simulink model "New_Control_Law"  (R2014a)
settings: configuration reference "AR_Drone_ConfigSet" (kept outside this file)
undefined symbols (not defined in the file or in its folder): Drone_StateModeType, sigbuilder_block
libraries: simulink x8, AR_Drone_2_Library x4
settings Model: SimulationMode=external  ExtModeTrigDuration=48000  Creator=nraman  LastModifiedBy=darenlee

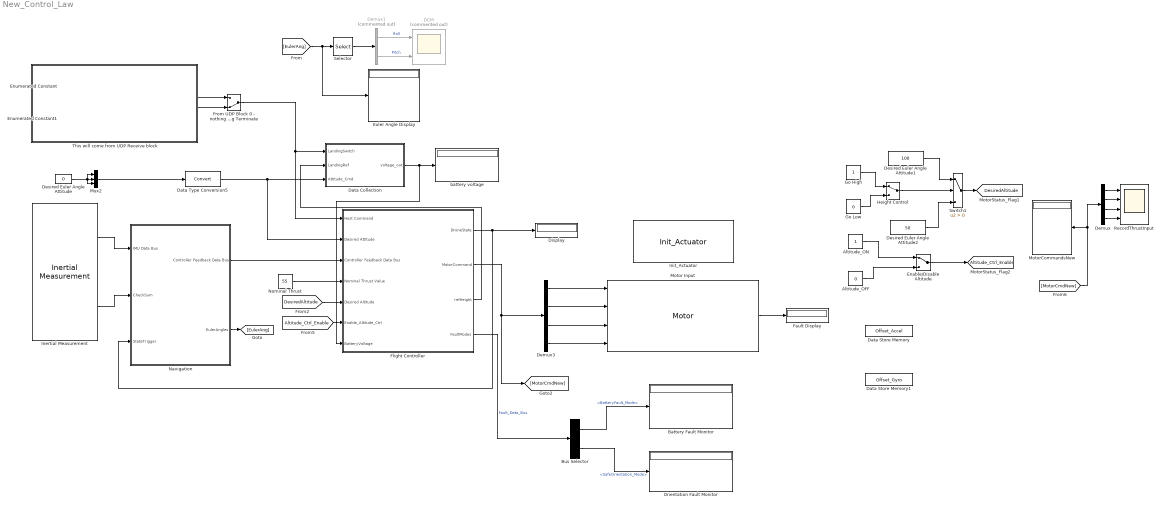
== system New_Control_Law ==
  Altitude_OFF : Constant  Value=0
  Altitude_ON : Constant
  Battery Fault Monitor : Display
  Bus Selector : BusSelector  OutputSignals=BatteryFault_Mode,SafeOrientation_Mode
  DCM : Scope  Commented=on  NumInputPorts=2
      settings: TimeRange=18.24617860016089  YMin=-20~-0.6  YMax=30~0.1  SaveName=EulerAngles
  Data Collection : Subsystem
  Data Store Memory : DataStoreMemory  DataStoreName=Offset_Accel  ReadBeforeWriteMsg=warning  WriteAfterWriteMsg=warning  WriteAfterReadMsg=warning  InitialValue=[0 0]  OutDataTypeStr=double
  Data Store Memory1 : DataStoreMemory  DataStoreName=Offset_Gyro  ReadBeforeWriteMsg=warning  WriteAfterWriteMsg=warning  WriteAfterReadMsg=warning  InitialValue=[0 0 0]  OutDataTypeStr=double
  Data Type Conversion5 : DataTypeConversion
  Demux : Demux
  Demux1 : Demux  Commented=on  Outputs=2
  Demux3 : Demux
  Desired Euler Angle Attitude : Constant  Value=0
  Desired Euler Angle Attitude1 : Constant  Value=100
  Desired Euler Angle Attitude2 : Constant  Value=50
  Display : Display
  Enable/Disable Altitude : ManualSwitch
  Enumerated Constant : simulink/Sources/Enumerated Constant  OutDataTypeStr=Enum: Drone_StateModeType  Value=Drone_StateModeType.Controlled_Flight  SampleTime=inf
  Enumerated Constant1 : simulink/Sources/Enumerated Constant  OutDataTypeStr=Enum: Drone_StateModeType  Value=Drone_StateModeType.Landing_Sequence  SampleTime=inf
  Euler Angle Display : Display
  Fault Display : Display
  Flight Controller : Subsystem
  "From UDP Block 0 - nothing 1 - Initialize 2 - take-off 3 - Land 4 - Landing Terminate " : ManualSwitch  CurrentSetting=0
  Go High : Constant
  Go Low : Constant  Value=0
  Height Control : ManualSwitch
  Inertial Measurement : AR_Drone_2_Library/Inertial Measurement  Ts=1/400
  Init_Actuator : AR_Drone_2_Library/Init_Actuator  ShowSpec=on
  Motor Input : AR_Drone_2_Library/Motor
  MotorCommandsNew : Display
  Mux2 : Mux  Inputs=3
  Navigation : Subsystem
  Nominal Thrust : Constant  Value=55
  Orientation Fault Monitor : Display
  RecordThrustInput : Scope  NumInputPorts=4
      settings: TimeRange=44.32823813354787  YMin=20~20~-5~-5  YMax=85~90~5~5  SaveName=Control_Input
  Selector : Selector  InputPortWidth=3  Indices=[1 2]
  Switch1 : Switch  Criteria=u2 > Threshold
  This will come from UDP Receive block : Subsystem
  battery voltage : Display
  tag scope: Altitude_Ctrl_Enable=global, DesiredAltitude=global
  wires:
  Motor Input/1 -> Fault Display/1
  Data Collection/1(voltage_out) -> Flight Controller/7(BatteryVoltage), battery voltage/1
  Mux2/1 -> Data Type Conversion5/1
  Demux3/1 -> Motor Input/1
  Demux3/2 -> Motor Input/2
  Demux3/3 -> Motor Input/3
  Demux3/4 -> Motor Input/4
  Inertial Measurement/1 -> Navigation/1(IMU Data Bus)
  Inertial Measurement/2 -> Navigation/2(CheckSum)
  Data Type Conversion5/1 -> Flight Controller/2(Desired Attitude), Data Collection/3(Attitude_Cmd)
  Nominal Thrust/1 -> Flight Controller/4(Nominal Thrust Value)
  Navigation/1(Controller Feedback Data Bus) -> Flight Controller/3(Controller Feedback Data Bus)
  Navigation/2(EulerAngles) -> [EulerAng]
  Go High/1 -> Height Control/1
  Go Low/1 -> Height Control/2
  Height Control/1 -> Switch1/2
  Desired Euler Angle Attitude1/1 -> Switch1/1
  Desired Euler Angle Attitude2/1 -> Switch1/3
  Switch1/1 -> [DesiredAltitude]
  [DesiredAltitude] -> Flight Controller/5(Desired Altitude)
  [Altitude_Ctrl_Enable] -> Flight Controller/6(Enable_Altitude_Ctrl)
  Altitude_ON/1 -> Enable/Disable Altitude/1
  Altitude_OFF/1 -> Enable/Disable Altitude/2
  Enable/Disable Altitude/1 -> [Altitude_Ctrl_Enable]
  Enumerated Constant1/1 -> "From UDP Block 0 - nothing 1 - Initialize 2 - take-off 3 - Land 4 - Landing Terminate "/2
  "From UDP Block 0 - nothing 1 - Initialize 2 - take-off 3 - Land 4 - Landing Terminate "/1 -> Flight Controller/1(Host Command), Data Collection/1(LandingSwitch)
  Flight Controller/1(DroneState) -> Navigation/3(StateTrigger), Display/1
  Demux1/1 -> DCM/1  "Roll"
  Demux1/2 -> DCM/2  "Pitch"
  [EulerAng] -> Selector/1, Euler Angle Display/1
  Selector/1 -> Demux1/1
  Enumerated Constant/1 -> "From UDP Block 0 - nothing 1 - Initialize 2 - take-off 3 - Land 4 - Landing Terminate "/1
  Flight Controller/3(refHeight) -> Data Collection/2(LandingRef)
  [MotorCmdNew] -> MotorCommandsNew/1, Demux/1
  Demux/1 -> RecordThrustInput/1
  Demux/2 -> RecordThrustInput/2
  Demux/3 -> RecordThrustInput/3
  Demux/4 -> RecordThrustInput/4
  Flight Controller/2(MotorCommand) -> Demux3/1, [MotorCmdNew]
  Desired Euler Angle Attitude/1 -> Mux2/3, Mux2/2, Mux2/1
  Flight Controller/4(FaultModes) -> Bus Selector/1  "Fault_Data_Bus"
  Bus Selector/1 -> Battery Fault Monitor/1  "<BatteryFault_Mode>"
  Bus Selector/2 -> Orientation Fault Monitor/1  "<SafeOrientation_Mode>"

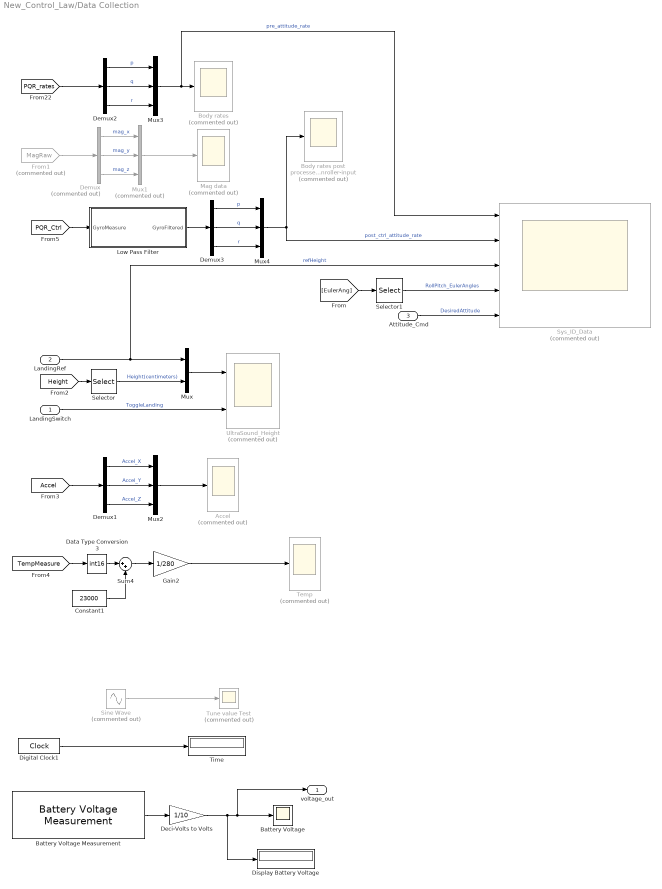
== system New_Control_Law/Data Collection ==
  LandingSwitch : Inport
  LandingRef : Inport  Port=2
  Attitude_Cmd : Inport  Port=3
  Accel : Scope  Commented=on
      settings: ShowLegends=on  TimeRange=100  YMin=1850  YMax=2750  SaveName=Accel
  Battery Voltage : Scope
      settings: YMin=11.935  YMax=12.005  SaveName=RecordedBattery
  Battery Voltage Measurement : AR_Drone_2_Library/Battery Voltage Measurement  SFunctionSpec=void BatteryMeasure_step(single y1[1])  SampleTime=1/400
  Body rates : Scope  Commented=on
      settings: ShowLegends=on  TimeRange=90  YMin=-1000  YMax=1200  SaveName=Gyro
  Body rates post processed - pre-conroller-input : Scope  Commented=on
      settings: ShowLegends=on  TimeRange=90  YMin=-1000  YMax=1200  SaveName=Gyro_PostProcessed
  Constant1 : Constant  Value=23000  OutDataTypeStr=int16
  Data Type Conversion3 : DataTypeConversion  OutDataTypeStr=int16
  Deci-Volts to Volts : Gain  Gain=1/10
  Demux : Demux  Commented=on  Outputs=3
  Demux1 : Demux  Outputs=3
  Demux2 : Demux  Outputs=3
  Demux3 : Demux  Outputs=3
  Digital Clock1 : DigitalClock  SampleTime=0.1
  Display Battery Voltage : Display
  From1 : From  Commented=on  GotoTag=MagRaw  TagVisibility=global
  Gain2 : Gain  Gain=1/280  OutDataTypeStr=double
  Low Pass Filter : Subsystem
  Mag data : Scope  Commented=on
      settings: ShowLegends=on  TimeRange=100  YMin=-15  YMax=50  SaveName=MagData
  Mux : Mux  Inputs=2
  Mux1 : Mux  Commented=on  Inputs=3
  Mux2 : Mux  Inputs=3
  Mux3 : Mux  Inputs=3
  Mux4 : Mux  Inputs=3
  Selector : Selector  InputPortWidth=2  Indices=[1]
  Selector1 : Selector  InputPortWidth=3  Indices=[1 2 3]
  Sine Wave : Sin  Commented=on  SineType=Sample based  Amplitude=6  Bias=-1  Samples=1000  SampleTime=0.01
  Sum4 : Sum  Inputs=|++
  Sys_ID_Data : Scope  Commented=on  NumInputPorts=5
      settings: ShowLegends=on  YMin=-5~-5~-5~-5~-5  YMax=5~5~5~5~5  SaveName=Sys_ID_Data_Record
  Temp : Scope  Commented=on
      settings: ShowLegends=on  TimeRange=100  YMin=47.83  YMax=48.03  SaveName=TempMeasure
  Time : Display
  Tune value Test : Scope  Commented=on
      settings: YMin=0.25  SaveName=UltraSound_Measure2
  UltraSound_Height : Scope  Commented=on  NumInputPorts=2
      settings: ShowLegends=on  TimeRange=1  YMin=0~-2  YMax=140~2  SaveName=UltrasoundHeight
  voltage_out : Outport
  wires:
  Sine Wave/1 -> Tune value Test/1
  Digital Clock1/1 -> Time/1
  From1/1 -> Demux/1
  Demux/1 -> Mux1/1  "mag_x"
  Demux/2 -> Mux1/2  "mag_y"
  Demux/3 -> Mux1/3  "mag_z"
  Mux1/1 -> Mag data/1
  Demux2/1 -> Mux3/1  "p"
  Demux2/2 -> Mux3/2  "q"
  Demux2/3 -> Mux3/3  "r"
  [PQR_rates] -> Demux2/1
  [Height] -> Selector/1
  Demux1/1 -> Mux2/1  "Accel_X"
  Demux1/2 -> Mux2/2  "Accel_Y"
  Mux2/1 -> Accel/1
  Demux1/3 -> Mux2/3  "Accel_Z"
  [Accel] -> Demux1/1
  Battery Voltage Measurement/1 -> Deci-Volts to Volts/1
  Deci-Volts to Volts/1 -> Display Battery Voltage/1, voltage_out/1, Battery Voltage/1
  Data Type Conversion3/1 -> Sum4/1
  Constant1/1 -> Sum4/2
  Sum4/1 -> Gain2/1
  Gain2/1 -> Temp/1
  [TempMeasure] -> Data Type Conversion3/1
  LandingSwitch/1 -> UltraSound_Height/2  "ToggleLanding"
  LandingRef/1 -> Mux/1, Sys_ID_Data/3  "refHeight"
  Mux/1 -> UltraSound_Height/1
  Selector/1 -> Mux/2  "Height(centimeters)"
  Demux3/1 -> Mux4/1  "p"
  Demux3/2 -> Mux4/2  "q"
  Demux3/3 -> Mux4/3  "r"
  [PQR_Ctrl] -> Low Pass Filter/1(GyroMeasure)
  Low Pass Filter/1(GyroFiltered) -> Demux3/1
  Mux4/1 -> Body rates post processed - pre-conroller-input/1, Sys_ID_Data/2  "post_ctrl_attitude_rate"
  Mux3/1 -> Sys_ID_Data/1, Body rates/1  "pre_attitude_rate"
  [EulerAng] -> Selector1/1
  Selector1/1 -> Sys_ID_Data/4  "RollPitch_EulerAngles"
  Attitude_Cmd/1 -> Sys_ID_Data/5  "DesiredAttitude"

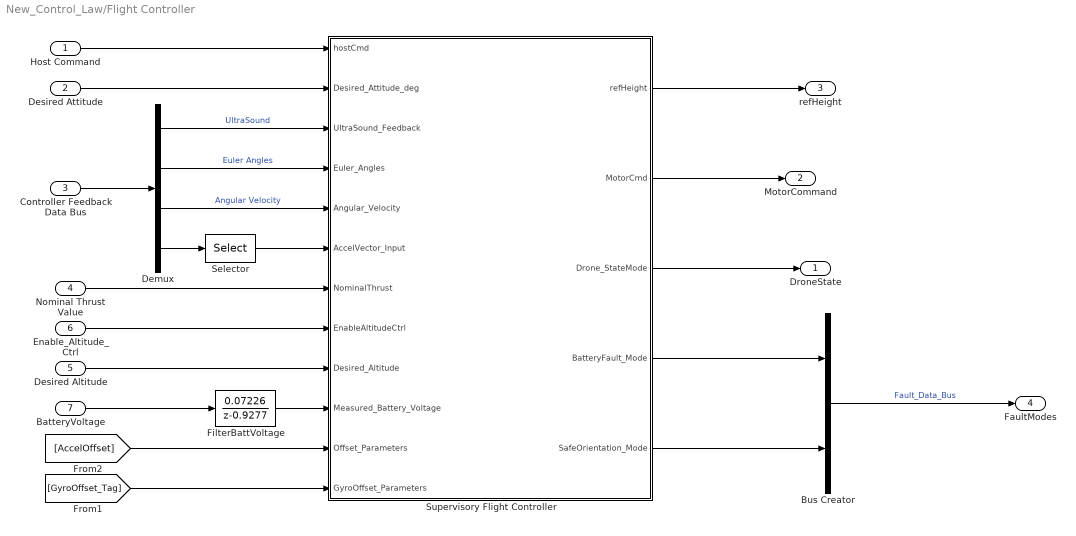
== system New_Control_Law/Flight Controller ==
  Host Command : Inport
  Desired Attitude : Inport  Port=2
  Controller Feedback Data Bus : Inport  Port=3
  Nominal Thrust Value : Inport  Port=4
  Desired Altitude : Inport  Port=5
  Enable_Altitude_Ctrl : Inport  Port=6
  BatteryVoltage : Inport  Port=7
  Bus Creator : BusCreator  Inputs=2
  Demux : Demux  Outputs=[2 3 3 3]
  FilterBattVoltage : DiscreteTransferFcn  Numerator=[ 0.07226]  Denominator=[1 -0.9277]  SampleTime=1/400
  Selector : Selector  InputPortWidth=3  Indices=[3]
  Supervisory Flight Controller : Stateflow chart  TreatAsAtomicUnit=on
  DroneState : Outport
  MotorCommand : Outport  Port=2
  refHeight : Outport  Port=3
  FaultModes : Outport  Port=4
  wires:
  Supervisory Flight Controller/2(MotorCmd) -> MotorCommand/1
  Desired Attitude/1 -> Supervisory Flight Controller/2(Desired_Attitude_deg)
  Desired Altitude/1 -> Supervisory Flight Controller/9(Desired_Altitude)
  Supervisory Flight Controller/3(" Drone_StateMode") -> DroneState/1
  Host Command/1 -> Supervisory Flight Controller/1(hostCmd)
  Demux/1 -> Supervisory Flight Controller/3(UltraSound_Feedback)  "UltraSound"
  Demux/2 -> Supervisory Flight Controller/4(Euler_Angles)  "Euler Angles"
  Demux/3 -> Supervisory Flight Controller/5(Angular_Velocity)  "Angular Velocity"
  Nominal Thrust Value/1 -> Supervisory Flight Controller/7(NominalThrust)
  Controller Feedback Data Bus/1 -> Demux/1
  Enable_Altitude_Ctrl/1 -> Supervisory Flight Controller/8(EnableAltitudeCtrl)
  [AccelOffset] -> Supervisory Flight Controller/11(Offset_Parameters)
  Supervisory Flight Controller/1(refHeight) -> refHeight/1
  [GyroOffset_Tag] -> Supervisory Flight Controller/12(GyroOffset_Parameters)
  BatteryVoltage/1 -> FilterBattVoltage/1
  FilterBattVoltage/1 -> Supervisory Flight Controller/10(Measured_Battery_Voltage)
  Demux/4 -> Selector/1
  Selector/1 -> Supervisory Flight Controller/6(AccelVector_Input)
  Supervisory Flight Controller/4(" BatteryFault_Mode") -> Bus Creator/1
  Supervisory Flight Controller/5(" SafeOrientation_Mode") -> Bus Creator/2
  Bus Creator/1 -> FaultModes/1  "Fault_Data_Bus"

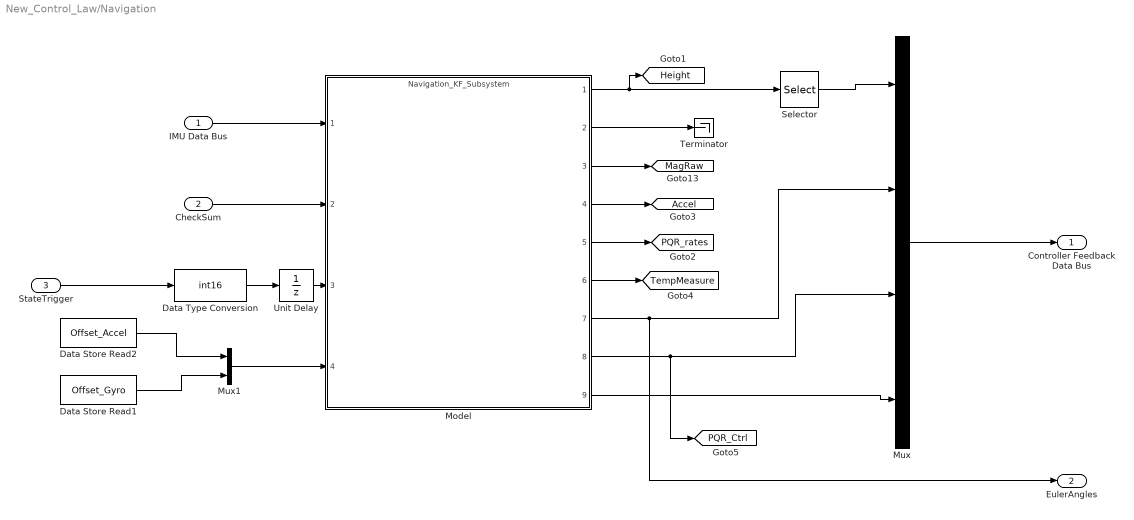
== system New_Control_Law/Navigation ==
  IMU Data Bus : Inport
  CheckSum : Inport  Port=2
  StateTrigger : Inport  Port=3  OutDataTypeStr=Enum: Drone_StateModeType
  Data Store Read1 : DataStoreRead  DataStoreName=Offset_Gyro
  Data Store Read2 : DataStoreRead  DataStoreName=Offset_Accel
  Data Type Conversion : DataTypeConversion  OutDataTypeStr=int16
  Model : ModelReference  ModelNameDialog=Navigation_KF_Subsystem.slx  SimulationMode=Normal  ModelReferenceVersion=1.15  CopyOfModelName=Navigation_KF_Subsystem.slx  DefaultDataLogging=on
  Mux : Mux
  Mux1 : Mux  Inputs=2
  Selector : Selector  InputPortWidth=2  Indices=[1 2]
  Terminator : Terminator
  Unit Delay : UnitDelay  SampleTime=-1
  Controller Feedback Data Bus : Outport
  EulerAngles : Outport  Port=2
  tag scope: Accel=global, Height=global, MagRaw=global, PQR_Ctrl=global, PQR_rates=global, TempMeasure=global
  wires:
  IMU Data Bus/1 -> Model/1
  CheckSum/1 -> Model/2
  Model/7 -> Mux/2, EulerAngles/1
  Model/1 -> [Height], Selector/1
  Model/8 -> [PQR_Ctrl], Mux/3
  Mux/1 -> Controller Feedback Data Bus/1
  Selector/1 -> Mux/1
  Model/2 -> Terminator/1
  Model/6 -> [TempMeasure]
  Model/5 -> [PQR_rates]
  Model/4 -> [Accel]
  Model/3 -> [MagRaw]
  StateTrigger/1 -> Data Type Conversion/1
  Model/9 -> Mux/4
  Data Store Read2/1 -> Mux1/1
  Mux1/1 -> Model/4
  Data Store Read1/1 -> Mux1/2
  Data Type Conversion/1 -> Unit Delay/1
  Unit Delay/1 -> Model/3

== system New_Control_Law/This will come from UDP Receive block ==

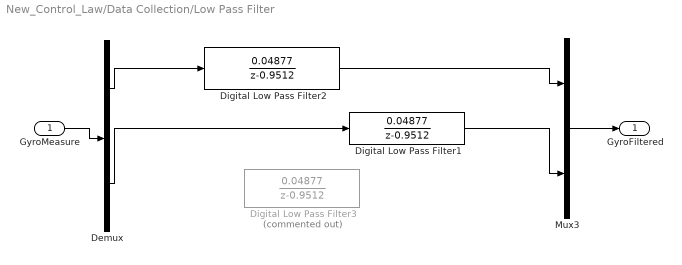
== system New_Control_Law/Data Collection/Low Pass Filter ==
  GyroMeasure : Inport
  Demux : Demux  Outputs=2
  Digital Low Pass Filter1 : DiscreteTransferFcn  Numerator=[0.04877]  Denominator=[1 -0.9512]  OutDataTypeStr=int16
  Digital Low Pass Filter2 : DiscreteTransferFcn  Numerator=[0.04877]  Denominator=[1 -0.9512]  OutDataTypeStr=int16
  Digital Low Pass Filter3 : DiscreteTransferFcn  Commented=on  Numerator=[0.04877]  Denominator=[1 -0.9512]  OutDataTypeStr=int16
  Mux3 : Mux  Inputs=2
  GyroFiltered : Outport
  wires:
  Mux3/1 -> GyroFiltered/1
  Demux/1 -> Digital Low Pass Filter2/1
  GyroMeasure/1 -> Demux/1
  Demux/2 -> Digital Low Pass Filter1/1
  Digital Low Pass Filter2/1 -> Mux3/1
  Digital Low Pass Filter1/1 -> Mux3/2

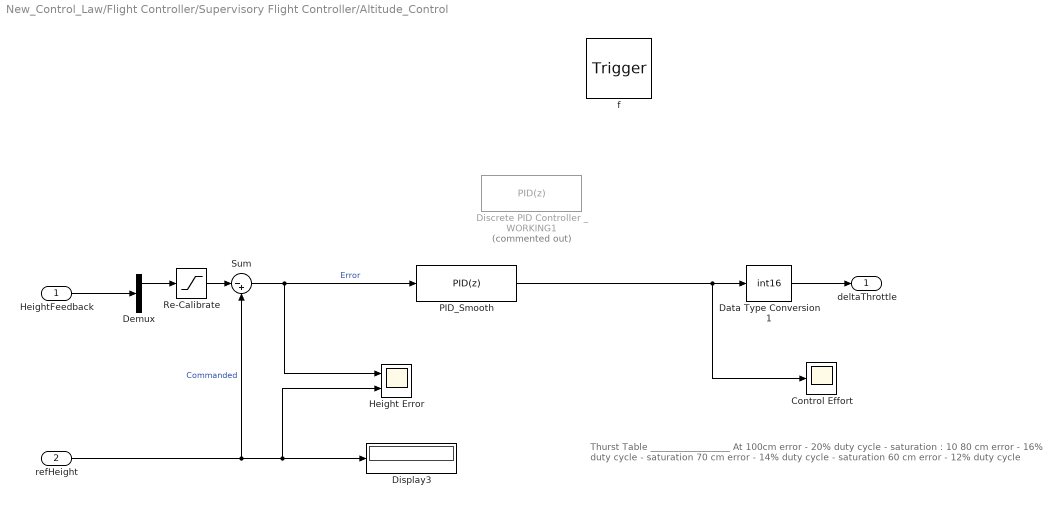
== system New_Control_Law/Flight Controller/Supervisory Flight Controller/Altitude_Control ==
  note: Thurst Table
      | _________________
      | At 100cm error  - 20% duty cycle - saturation : 10
      | 80 cm error - 16% duty cycle - saturation
      | 70 cm error - 14% duty cycle - saturation
      | 60 cm error - 12% duty cycle
  HeightFeedback : Inport  OutDataTypeStr=double  PortDimensions=2
  refHeight : Inport  Port=2  OutDataTypeStr=double  PortDimensions=1
  f : TriggerPort  TriggerType=function-call
      settings: CopyFcn=Stateflow.SLINSF.SimulinkMan.removeBlockPreDeleteFcn  PreDeleteFcn=Stateflow.SLINSF.SimulinkMan.unsafePredeleteFcn
  Control Effort : Scope
      settings: YMin=8.735  YMax=8.7875  SaveName=ScopeData3
  Data Type Conversion1 : DataTypeConversion  OutDataTypeStr=int16
  Demux : Demux  Outputs=2
  Discrete PID Controller _ WORKING1 : simulink/Continuous/PID Controller  Commented=on  Controller=PID  TimeDomain=Discrete-time  SampleTime=-1  IntegratorMethod=Forward Euler  FilterMethod=Forward Euler  Form=Parallel  P=0.387369235850492*0.7  I=0.018136*4  D=0.819231727791919*0.15  N=12.5907330811849  InitialConditionSource=internal  InitialConditionForIntegrator=0  InitialConditionForFilter=0  ExternalReset=none  LimitOutput=on  UpperSaturationLimit=20  LowerSaturationLimit=-20  LinearizeAsGain=off  AntiWindupMode=clamping  Kb=1  TrackingMode=off  Kt=1  PParamMin=[]  PParamMax=[]  IParamMin=[]  IParamMax=[]  DParamMin=[]  DParamMax=[]  NParamMin=[]  NParamMax=[]  KbParamMin=[]  KbParamMax=[]  KtParamMin=[]  KtParamMax=[]  POutMin=[]  POutMax=[]  IOutMin=[]  IOutMax=[]  DOutMin=[]  DOutMax=[]  NOutMin=[]  NOutMax=[]  KbOutMin=[]  KbOutMax=[]  KtOutMin=[]  KtOutMax=[]  IntegratorOutMin=[]  IntegratorOutMax=[]  FilterOutMin=[]  FilterOutMax=[]  SumOutMin=[]  SumOutMax=[]  SumI1OutMin=[]  SumI1OutMax=[]  SumI2OutMin=[]  SumI2OutMax=[]  SumI3OutMin=[]  SumI3OutMax=[]  SumDOutMin=[]  SumDOutMax=[]  SaturationOutMin=[]  SaturationOutMax=[]  IntegratorContinuousStateAttributes=''  IntegratorStateMustResolveToSignalObject=off  IntegratorRTWStateStorageClass=Auto  FilterContinuousStateAttributes=''  FilterStateMustResolveToSignalObject=off  FilterRTWStateStorageClass=Auto
  Display3 : Display
  Height Error : Scope  NumInputPorts=2
      settings: ShowLegends=on  YMin=-0.1075~-5  YMax=-0.08~5  SaveName=ScopeData13
  PID_Smooth : simulink/Continuous/PID Controller  Controller=PID  TimeDomain=Discrete-time  SampleTime=-1  IntegratorMethod=Forward Euler  FilterMethod=Forward Euler  Form=Parallel  P=0.387369235850492*0.7  I=0.018136*4  D=0.819231727791919*0.15  N=12.5907330811849  InitialConditionSource=internal  InitialConditionForIntegrator=0  InitialConditionForFilter=0  ExternalReset=none  LimitOutput=on  UpperSaturationLimit=20  LowerSaturationLimit=-20  LinearizeAsGain=off  AntiWindupMode=clamping  Kb=1  TrackingMode=off  Kt=1  PParamMin=[]  PParamMax=[]  IParamMin=[]  IParamMax=[]  DParamMin=[]  DParamMax=[]  NParamMin=[]  NParamMax=[]  KbParamMin=[]  KbParamMax=[]  KtParamMin=[]  KtParamMax=[]  POutMin=[]  POutMax=[]  IOutMin=[]  IOutMax=[]  DOutMin=[]  DOutMax=[]  NOutMin=[]  NOutMax=[]  KbOutMin=[]  KbOutMax=[]  KtOutMin=[]  KtOutMax=[]  IntegratorOutMin=[]  IntegratorOutMax=[]  FilterOutMin=[]  FilterOutMax=[]  SumOutMin=[]  SumOutMax=[]  SumI1OutMin=[]  SumI1OutMax=[]  SumI2OutMin=[]  SumI2OutMax=[]  SumI3OutMin=[]  SumI3OutMax=[]  SumDOutMin=[]  SumDOutMax=[]  SaturationOutMin=[]  SaturationOutMax=[]  IntegratorContinuousStateAttributes=''  IntegratorStateMustResolveToSignalObject=off  IntegratorRTWStateStorageClass=Auto  FilterContinuousStateAttributes=''  FilterStateMustResolveToSignalObject=off  FilterRTWStateStorageClass=Auto
  Re-Calibrate : Saturate  UpperLimit=200  LowerLimit=0  OutMin=0  OutMax=200
      settings: AttributesFormatString=|
      | Upper: %<UpperLimit>
      | Lower %<LowerLimit>
  Sum : Sum  Inputs=|-+
  deltaThrottle : Outport  OutDataTypeStr=int16
  wires:
  refHeight/1 -> Sum/2, Height Error/2, Display3/1  "Commanded"
  PID_Smooth/1 -> Control Effort/1, Data Type Conversion1/1
  Data Type Conversion1/1 -> deltaThrottle/1
  HeightFeedback/1 -> Demux/1
  Demux/1 -> Re-Calibrate/1
  Sum/1 -> PID_Smooth/1, Height Error/1  "Error"
  Re-Calibrate/1 -> Sum/1

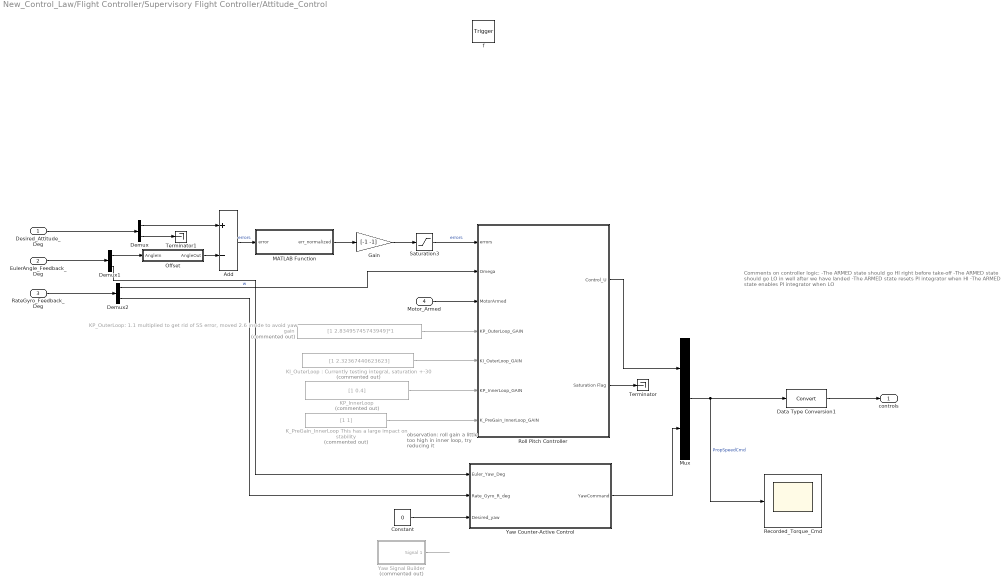
== system New_Control_Law/Flight Controller/Supervisory Flight Controller/Attitude_Control ==
  note: observation:
      | roll gain a little
      | too high in inner
      | loop, try reducing it
  note: Comments on controller logic:
      | -The ARMED state should go HI right before take-off
      | -The  ARMED state should go LO in well after we have landed
      | -The ARMED state resets PI integrator when HI
      | -The ARMED state enables PI integrator when LO
  Desired_Attitude_Deg : Inport  OutDataTypeStr=double  PortDimensions=3
  EulerAngle_Feedback_Deg : Inport  Port=2  OutDataTypeStr=double  PortDimensions=3
  RateGyro_Feedback_Deg : Inport  Port=3  OutDataTypeStr=double  PortDimensions=3
  Motor_Armed : Inport  Port=4  OutDataTypeStr=double  PortDimensions=1
  f : TriggerPort  TriggerType=function-call
      settings: CopyFcn=Stateflow.SLINSF.SimulinkMan.removeBlockPreDeleteFcn  PreDeleteFcn=Stateflow.SLINSF.SimulinkMan.unsafePredeleteFcn
  Add : Sum  Inputs=+-  AccumDataTypeStr=single  OutDataTypeStr=single
  Constant : Constant  Value=0
  Data Type Conversion1 : DataTypeConversion
  Demux : Demux  Outputs=[2 1]
  Demux1 : Demux  Outputs=[2 1]
  Demux2 : Demux  Outputs=[2 1]
  Gain : Gain  Gain=[-1 -1]
  "KI_OuterLoop : Currently testing integral, saturation +-30" : Constant  Commented=on  Value=[1 2.32367440623623]
  KP_InnerLoop : Constant  Commented=on  Value=[1 0.4]
  "KP_OuterLoop: 1.1 multiplied to get rid of SS error, moved 2.6 inside to avoid yaw gain" : Constant  Commented=on  Value=[1 2.83495745743949]*1
  K_PreGain_InnerLoop This has a large impact on stability : Constant  Commented=on  Value=[1 1]
  MATLAB Function : MATLAB Function  TreatAsAtomicUnit=on
  Mux : Mux  Inputs=2
  Offset : Subsystem
  Recorded_Torque_Cmd : Scope
      settings: TimeRange=30  YMin=-30  YMax=30  SaveName=Toqrue_Input
  Roll Pitch Controller : Subsystem  TreatAsAtomicUnit=on
  Saturation3 : Saturate  UpperLimit=[25 25]  LowerLimit=[-25 -25]  OutDataTypeStr=single
      settings: AttributesFormatString=%<LowerLimit> to %<UpperLimit>
  Terminator : Terminator
  Terminator1 : Terminator
  Yaw Counter-Active Control : Subsystem
  "Yaw Signal Builder " : Subsystem  Tag=STV Subsys  Commented=on  LoadFcn=sigbuilder_block('load');  StartFcn=sigbuilder_block('start');  StopFcn=sigbuilder_block('stop');  ClipboardFcn=sigbuilder_block('clipboard');  mask(Sigbuilder block){}
      mask help: Simulink:masks:SigbuilderBlock_MD
      mask init:
      | if ~strcmp(get_param(bdroot(gcbh),'SimulationStatus'),'stopped') tuvar = sigbuilder_block('maskInit'); end
      settings: CopyFcn=sigbuilder_block('copy');  DeleteFcn=sigbuilder_block('delete');  ModelCloseFcn=sigbuilder_block('modelClose');  PreSaveFcn=sigbuilder_block('preSave');  PauseFcn=sigbuilder_block('pause');  ContinueFcn=sigbuilder_block('continue');  NameChangeFcn=sigbuilder_block('namechange');  OpenFcn=sigbuilder_block('open',[437.25 118.5 550.5 394.5 ]);  CloseFcn=sigbuilder_block('close');
      mask Display: plot(0, 0, 100, 100,[2, 2, 32, 32, 2], [68, 8, 8, 68, 68],[32, 2], [38, 38], [32, 19, 2],[53, 60, 44], [32, 17, 17, 2],[16, 16, 31, 31]);txt = getActiveGroup(gcbh);text(2, 100, txt,'verticalAlignment', 'top');
  controls : Outport  OutDataTypeStr=int16  PortDimensions=3  InitialOutput=0
  wires:
  Add/1 -> MATLAB Function/1(error)  "errors"
  Demux1/1 -> Offset/1(AngleIn)
  Demux2/1 -> Roll Pitch Controller/2(Omega)  "w"
  KP_InnerLoop/1 -> Roll Pitch Controller/6(KP_InnerLoop_GAIN)
  "KP_OuterLoop: 1.1 multiplied to get rid of SS error, moved 2.6 inside to avoid yaw gain"/1 -> Roll Pitch Controller/4(KP_OuterLoop_GAIN)
  K_PreGain_InnerLoop This has a large impact on stability/1 -> Roll Pitch Controller/7(K_PreGain_InnerLoop_GAIN)
  "KI_OuterLoop : Currently testing integral, saturation +-30"/1 -> Roll Pitch Controller/5(KI_OuterLoop_GAIN)
  Saturation3/1 -> Roll Pitch Controller/1(errors)  "errors"
  MATLAB Function/1(err_normalized) -> Gain/1
  Gain/1 -> Saturation3/1
  Roll Pitch Controller/2(Saturation Flag) -> Terminator/1
  Demux/1 -> Add/1
  Roll Pitch Controller/1(Control_U) -> Mux/1
  Demux/2 -> Terminator1/1
  Offset/1(AngleOut) -> Add/2
  Demux2/2 -> Yaw Counter-Active Control/2(Rate_Gyro_R_deg)
  Yaw Counter-Active Control/1(YawCommand) -> Mux/2
  Desired_Attitude_Deg/1 -> Demux/1
  EulerAngle_Feedback_Deg/1 -> Demux1/1
  RateGyro_Feedback_Deg/1 -> Demux2/1
  Motor_Armed/1 -> Roll Pitch Controller/3(MotorArmed)
  Demux1/2 -> Yaw Counter-Active Control/1(Euler_Yaw_Deg)
  Data Type Conversion1/1 -> controls/1
  Mux/1 -> Data Type Conversion1/1, Recorded_Torque_Cmd/1  "PropSpeedCmd"
  "Yaw Signal Builder "/1(Signal 1) -> ?
  Constant/1 -> Yaw Counter-Active Control/3("Desired_yaw ")

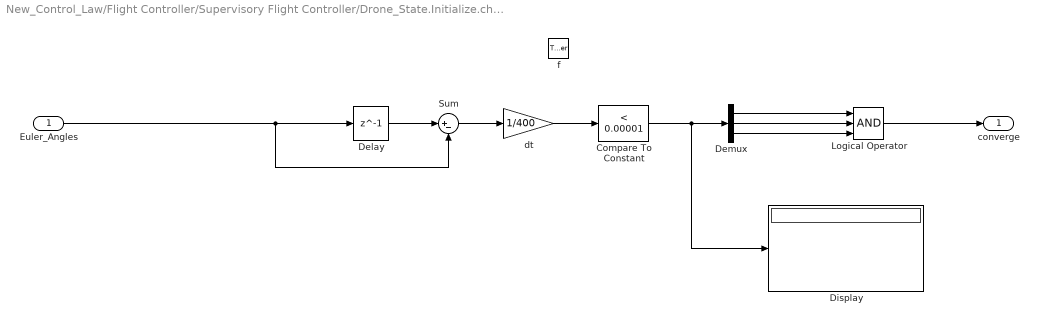
== system New_Control_Law/Flight Controller/Supervisory Flight Controller/Drone_State.Initialize.checkConvergence ==
  Euler_Angles : Inport  OutDataTypeStr=double  PortDimensions=3
  f : TriggerPort  TriggerType=function-call
      settings: CopyFcn=Stateflow.SLINSF.SimulinkMan.removeBlockPreDeleteFcn  PreDeleteFcn=Stateflow.SLINSF.SimulinkMan.unsafePredeleteFcn
  Compare To Constant : simulink/Logic and Bit Operations/Compare To Constant  relop=<  const=0.00001  OutDataTypeStr=boolean
  Delay : Delay  DelayLength=1  InitialCondition=inf
  Demux : Demux  Outputs=3
  Display : Display
  Logical Operator : Logic  Inputs=3  AllPortsSameDT=off  OutDataTypeStr=boolean
  Sum : Sum  Inputs=|+-
  dt : Gain  Gain=1/400
  converge : Outport
  wires:
  Euler_Angles/1 -> Sum/2, Delay/1
  Delay/1 -> Sum/1
  Sum/1 -> dt/1
  dt/1 -> Compare To Constant/1
  Compare To Constant/1 -> Display/1, Demux/1
  Logical Operator/1 -> converge/1
  Demux/1 -> Logical Operator/1
  Demux/2 -> Logical Operator/2
  Demux/3 -> Logical Operator/3

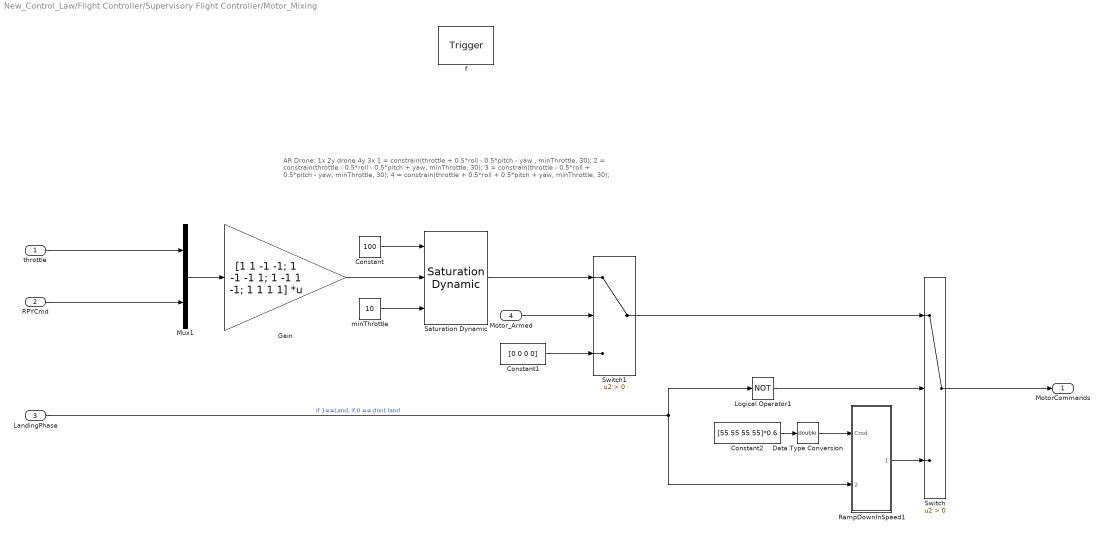
== system New_Control_Law/Flight Controller/Supervisory Flight Controller/Motor_Mixing ==
  note: AR Drone:
      |
      |   1x         2y
      |      drone
      |   4y         3x
      |
      |  1 = constrain(throttle + 0.5*roll - 0.5*pitch - yaw , minThrottle, 30);
      |  2 = constrain(throttle - 0.5*roll - 0.5*pitch + yaw, minThrottle, 30);
      |  3 = constrain(throttle - 0.5*roll + 0.5*pitch - yaw, minThrottle, 30);
      |  4 = constrain(throttle + 0.5*roll + 0.5*pitch + yaw, minThrottle, 30);
  throttle : Inport  OutDataTypeStr=int16  PortDimensions=1
  RPYCmd : Inport  Port=2  OutDataTypeStr=int16  PortDimensions=3
  LandingPhase : Inport  Port=3  OutDataTypeStr=double  PortDimensions=1
  Motor_Armed : Inport  Port=4  OutDataTypeStr=double  PortDimensions=1
  f : TriggerPort  TriggerType=function-call
      settings: CopyFcn=Stateflow.SLINSF.SimulinkMan.removeBlockPreDeleteFcn  PreDeleteFcn=Stateflow.SLINSF.SimulinkMan.unsafePredeleteFcn
  Constant : Constant  Value=100  OutDataTypeStr=int16  SampleTime=-1
  Constant1 : Constant  Value=[0 0 0 0]  OutDataTypeStr=int16
  Constant2 : Constant  Value=[55 55 55 55]*0.6
  Data Type Conversion : DataTypeConversion  OutDataTypeStr=double
  Gain : Gain  Gain=[1 1 -1 -1; 1 -1 -1 1; 1 -1 1 -1; 1 1 1 1]  Multiplication=Matrix(K*u)  ParamDataTypeStr=int16  OutDataTypeStr=int16
  Logical Operator1 : Logic  Operator=NOT  AllPortsSameDT=off  OutDataTypeStr=boolean
  Mux1 : Mux  Inputs=2
  RampDownInSpeed1 : MATLAB Function  TreatAsAtomicUnit=on
  Saturation Dynamic : simulink/Discontinuities/Saturation Dynamic  OutMin=[]  OutMax=[]  OutDataTypeStr=Inherit: Same as second input  OutDataType=fixdt(1, 16)  OutScaling=2^-10  DoSatur=off
  Switch : Switch  Criteria=u2 > Threshold
  Switch1 : Switch  Criteria=u2 > Threshold
  minThrottle : Constant  Value=10  OutDataTypeStr=int16
  MotorCommands : Outport  InitialOutput=0
  wires:
  RPYCmd/1 -> Mux1/2
  minThrottle/1 -> Saturation Dynamic/3
  Constant/1 -> Saturation Dynamic/1
  Mux1/1 -> Gain/1
  Gain/1 -> Saturation Dynamic/2
  throttle/1 -> Mux1/1
  Data Type Conversion/1 -> RampDownInSpeed1/1(Cmd)
  RampDownInSpeed1/1(motorCmd) -> Switch/3
  Constant2/1 -> Data Type Conversion/1
  LandingPhase/1 -> RampDownInSpeed1/2(stopCmd), Logical Operator1/1  "if 1==Land, if 0 == dont land"
  Switch/1 -> MotorCommands/1
  Logical Operator1/1 -> Switch/2
  Saturation Dynamic/1 -> Switch1/1
  Motor_Armed/1 -> Switch1/2
  Constant1/1 -> Switch1/3
  Switch1/1 -> Switch/1

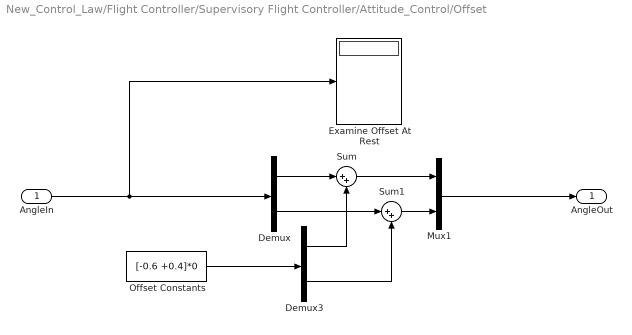
== system New_Control_Law/Flight Controller/Supervisory Flight Controller/Attitude_Control/Offset ==
  AngleIn : Inport
  Demux : Demux  Outputs=2
  Demux3 : Demux  Outputs=2
  Examine Offset At Rest : Display
  Mux1 : Mux  Inputs=2
  Offset Constants : Constant  Value=[-0.6 +0.4]*0  OutDataTypeStr=single
  Sum : Sum  Inputs=|++
  Sum1 : Sum  Inputs=|++
  AngleOut : Outport
  wires:
  Mux1/1 -> AngleOut/1
  Sum/1 -> Mux1/1
  Sum1/1 -> Mux1/2
  Demux/2 -> Sum1/1
  AngleIn/1 -> Examine Offset At Rest/1, Demux/1
  Demux3/2 -> Sum1/2
  Demux3/1 -> Sum/2
  Demux/1 -> Sum/1
  Offset Constants/1 -> Demux3/1

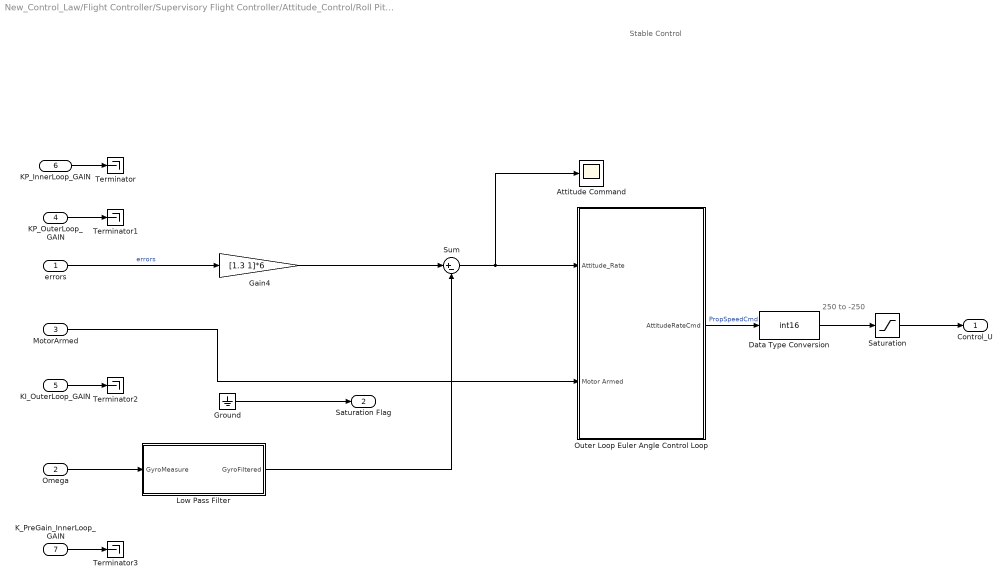
== system New_Control_Law/Flight Controller/Supervisory Flight Controller/Attitude_Control/Roll Pitch Controller ==
  note: 250 to -250
  note: Stable Control
  errors : Inport
  Omega : Inport  Port=2
  MotorArmed : Inport  Port=3
  KP_OuterLoop_GAIN : Inport  Port=4
  KI_OuterLoop_GAIN : Inport  Port=5
  KP_InnerLoop_GAIN : Inport  Port=6
  K_PreGain_InnerLoop_GAIN : Inport  Port=7
  Attitude Command : Scope
      settings: SaveName=AttitudeRateCtrl_Cmd
  Data Type Conversion : DataTypeConversion  OutDataTypeStr=int16  RndMeth=Nearest
  Gain4 : Gain  Gain=[1.3 1]*6
  Ground : Ground
  Low Pass Filter : Subsystem
  Outer Loop Euler Angle Control Loop : Subsystem
  Saturation : Saturate  UpperLimit=250  LowerLimit=-250  OutDataTypeStr=int16
      settings: AttributesFormatString=%<LowerLimit>\nto\n%<UpperLimit>
  Sum : Sum  Inputs=|+-
  Terminator{,1..3} (4 alike) : Terminator
  Control_U : Outport
  Saturation Flag : Outport  Port=2
  wires:
  Saturation/1 -> Control_U/1
  Data Type Conversion/1 -> Saturation/1
  Outer Loop Euler Angle Control Loop/1(AttitudeRateCmd) -> Data Type Conversion/1  "PropSpeedCmd"
  MotorArmed/1 -> Outer Loop Euler Angle Control Loop/2(Motor Armed)
  Ground/1 -> Saturation Flag/1
  Omega/1 -> Low Pass Filter/1(GyroMeasure)
  errors/1 -> Gain4/1  "errors"
  Sum/1 -> Attitude Command/1, Outer Loop Euler Angle Control Loop/1(Attitude_Rate)
  Gain4/1 -> Sum/1
  Low Pass Filter/1(GyroFiltered) -> Sum/2
  KP_InnerLoop_GAIN/1 -> Terminator/1
  KP_OuterLoop_GAIN/1 -> Terminator1/1
  KI_OuterLoop_GAIN/1 -> Terminator2/1
  K_PreGain_InnerLoop_GAIN/1 -> Terminator3/1

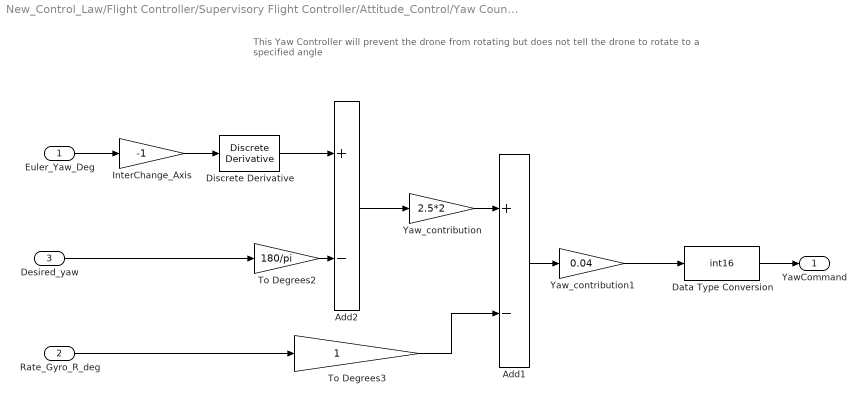
== system New_Control_Law/Flight Controller/Supervisory Flight Controller/Attitude_Control/Yaw Counter-Active Control ==
  note: This Yaw Controller will prevent the drone from
      | rotating but does not tell the drone to rotate to a specified angle
  Euler_Yaw_Deg : Inport
  Rate_Gyro_R_deg : Inport  Port=2
  "Desired_yaw " : Inport  Port=3
  Add1 : Sum  Inputs=+-  AccumDataTypeStr=single  OutDataTypeStr=single
  Add2 : Sum  Inputs=+-  AccumDataTypeStr=single  OutDataTypeStr=single
  Data Type Conversion : DataTypeConversion  OutDataTypeStr=int16
  Discrete Derivative : simulink/Discrete/Discrete Derivative  gainval=1.0  ICPrevScaledInput=0.0  InputProcessing=Inherited  OutMin=[]  OutMax=[]  OutDataType=fixdt(1, 16)  OutScaling=2^-10  DoSatur=off
  InterChange_Axis : Gain  Gain=-1  ParamDataTypeStr=single  OutDataTypeStr=single
      settings: AttributesFormatString=%<Gain>
  To Degrees2 : Gain  Gain=180/pi  ParamDataTypeStr=single  OutDataTypeStr=single
      settings: AttributesFormatString=%<Gain>
  To Degrees3 : Gain  ParamDataTypeStr=single  OutDataTypeStr=single
      settings: AttributesFormatString=%<Gain>
  Yaw_contribution : Gain  Gain=2.5*2  ParamDataTypeStr=single  OutDataTypeStr=single
      settings: AttributesFormatString=%<Gain>
  Yaw_contribution1 : Gain  Gain=0.04  ParamDataTypeStr=single  OutDataTypeStr=single
      settings: AttributesFormatString=%<Gain>
  YawCommand : Outport
  wires:
  Yaw_contribution1/1 -> Data Type Conversion/1
  To Degrees3/1 -> Add1/2
  Euler_Yaw_Deg/1 -> InterChange_Axis/1
  Add1/1 -> Yaw_contribution1/1
  Yaw_contribution/1 -> Add1/1
  Add2/1 -> Yaw_contribution/1
  InterChange_Axis/1 -> Discrete Derivative/1
  Discrete Derivative/1 -> Add2/1
  To Degrees2/1 -> Add2/2
  "Desired_yaw "/1 -> To Degrees2/1
  Rate_Gyro_R_deg/1 -> To Degrees3/1
  Data Type Conversion/1 -> YawCommand/1

== system New_Control_Law/Flight Controller/Supervisory Flight Controller/Attitude_Control/Yaw Signal Builder  ==
  Demux : Demux  Tag=STV Demux  Outputs=1
  FromWs : FromWorkspace  Tag=STV FromWs  VariableName=tuvar
      SigBuilderData=|
      | common.afterFinalStr = 'Extrapolate'
      | common.sampleTime = '-1'
      | dataSet.timeRange = [0 20]
      | dataSet.name = 'Group 1'
      | sbobj.Groups.Name = 'Group 1'
      | sbobj.Groups.Signals.Name = 'Signal 1'
      | sbobj.Groups.Signals.XData = [0 10 10 12.5 12.5 15 15 20]
      | sbobj.Groups.Signals.YData = [0 0 2 2 -2 -2 0 0]
      | sbobj.Groups.TimeRange = [0 20]
  Signal 1 : Outport  Tag=STV Outport
  wires:
  Demux/1 -> Signal 1/1
  FromWs/1 -> Demux/1

== system New_Control_Law/Flight Controller/Supervisory Flight Controller/Attitude_Control/Roll Pitch Controller/Low Pass Filter ==
  GyroMeasure : Inport
  Demux : Demux  Outputs=2
  Digital Low Pass Filter1 : DiscreteTransferFcn  Numerator=[0.04877]  Denominator=[1 -0.9512]  OutDataTypeStr=int16
  Digital Low Pass Filter2 : DiscreteTransferFcn  Numerator=[0.04877]  Denominator=[1 -0.9512]  OutDataTypeStr=int16
  Digital Low Pass Filter3 : DiscreteTransferFcn  Commented=on  Numerator=[0.04877]  Denominator=[1 -0.9512]  OutDataTypeStr=int16
  Mux3 : Mux  Inputs=2
  GyroFiltered : Outport
  wires:
  Mux3/1 -> GyroFiltered/1
  Demux/1 -> Digital Low Pass Filter2/1
  GyroMeasure/1 -> Demux/1
  Demux/2 -> Digital Low Pass Filter1/1
  Digital Low Pass Filter2/1 -> Mux3/1
  Digital Low Pass Filter1/1 -> Mux3/2

== system New_Control_Law/Flight Controller/Supervisory Flight Controller/Attitude_Control/Roll Pitch Controller/Outer Loop Euler Angle Control Loop ==
  Attitude_Rate : Inport
  Motor Armed : Inport  Port=2
  Logical Operator : Logic  Operator=NOT  AllPortsSameDT=off  OutDataTypeStr=boolean
  PID Controller : simulink/Continuous/PID Controller  Controller=PID  TimeDomain=Discrete-time  SampleTime=-1  IntegratorMethod=Forward Euler  FilterMethod=Forward Euler  Form=Parallel  P=0.10084  I=0.13631  D=-0.011755  N=5  InitialConditionSource=internal  InitialConditionForIntegrator=0  InitialConditionForFilter=0  ExternalReset=level  LimitOutput=on  UpperSaturationLimit=30  LowerSaturationLimit=-30  LinearizeAsGain=on  AntiWindupMode=clamping  Kb=1  TrackingMode=off  Kt=1  PParamMin=[]  PParamMax=[]  IParamMin=[]  IParamMax=[]  DParamMin=[]  DParamMax=[]  NParamMin=[]  NParamMax=[]  KbParamMin=[]  KbParamMax=[]  KtParamMin=[]  KtParamMax=[]  POutMin=[]  POutMax=[]  IOutMin=[]  IOutMax=[]  DOutMin=[]  DOutMax=[]  NOutMin=[]  NOutMax=[]  KbOutMin=[]  KbOutMax=[]  KtOutMin=[]  KtOutMax=[]  IntegratorOutMin=[]  IntegratorOutMax=[]  FilterOutMin=[]  FilterOutMax=[]  SumOutMin=[]  SumOutMax=[]  SumI1OutMin=[]  SumI1OutMax=[]  SumI2OutMin=[]  SumI2OutMax=[]  SumI3OutMin=[]  SumI3OutMax=[]  SumDOutMin=[]  SumDOutMax=[]  SaturationOutMin=[]  SaturationOutMax=[]  IntegratorContinuousStateAttributes=''  IntegratorStateMustResolveToSignalObject=off  IntegratorRTWStateStorageClass=Auto  FilterContinuousStateAttributes=''  FilterStateMustResolveToSignalObject=off  FilterRTWStateStorageClass=Auto
  AttitudeRateCmd : Outport
  wires:
  PID Controller/1 -> AttitudeRateCmd/1  "AttitudeRateCmd"
  Motor Armed/1 -> Logical Operator/1
  Logical Operator/1 -> PID Controller/2
  Attitude_Rate/1 -> PID Controller/1

== stateflow chart New_Control_Law/Flight Controller/Supervisory Flight Controller ==
  state Fault_Check [parallel]
    settings: executionOrder=3
    state BatteryFault_Check [parallel]
      settings: executionOrder=1
      state BatteryNominal
        en:
        BatteryFault = 0;
        state Nominal
        note: Description:
            | This state will be responsible for the following
            |
            | - Automatically land the drone by forcing it to the land state when voltage is low
            | - Prevent drone from taking off if battery voltage is too low
        state EvaluateVoltageLevel
        state ChangeState
          en:
          BatteryFault = 1;
        EvaluateVoltageLevel -> Fault_Check.BatteryFault_Check.BatteryNominal.Nominal [order 1] : [Measured_Battery_Voltage>=10.1]
        Fault_Check.BatteryFault_Check.BatteryNominal.Nominal -> EvaluateVoltageLevel : [Measured_Battery_Voltage<10.1]
        (default) -> EvaluateVoltageLevel
        EvaluateVoltageLevel -> Fault_Check.BatteryFault_Check.BatteryNominal.ChangeState [order 2] : after(5,sec)
      state BatteryLow
        state ForceLanding
          en:
        (default) -> ForceLanding
      (default) -> BatteryNominal
      BatteryNominal -> BatteryLow : [BatteryFault==1]
    state UltraSoundwarning_Check [parallel]
      settings: executionOrder=2
    state SafeOrientation_Check [parallel]
      settings: executionOrder=3
      state UnsafeOrientation
        du:
        MotorArmed =0;
        LandingPhase = 0;
      state WaitForFlight
      state GravityVectorCheck
        en:
        OrientationFault = 0;
        note: Description:
            | This state will be responsible for the following
            |
            | - Automatically land the drone by forcing it to the land state when voltage is low
            | - Prevent drone from taking off if battery voltage is too low
        state Nominal
        state EvaluateGravityVector
        state ChangeState
          en:
          OrientationFault = 1;
        EvaluateGravityVector -> Fault_Check.SafeOrientation_Check.GravityVectorCheck.Nominal [order 1] : [AccelVector_Input<-0.05]
        Fault_Check.SafeOrientation_Check.GravityVectorCheck.Nominal -> EvaluateGravityVector : [AccelVector_Input>=0.05]
        (default) -> EvaluateGravityVector
        EvaluateGravityVector -> Fault_Check.SafeOrientation_Check.GravityVectorCheck.ChangeState [order 2] : after(0.01,sec)
      (default) -> WaitForFlight
      GravityVectorCheck -> WaitForFlight [order 2] : [in(Drone_State.WaitForHost)]
      GravityVectorCheck -> UnsafeOrientation [order 1] : [OrientationFault ==1]
      WaitForFlight -> GravityVectorCheck : [in(Drone_State.Controlled_Flight)]
  state Drone_State [parallel]
    settings: executionOrder=1
    state WaitForHost
      entry:
      reset_offset_calc = 0;
      MotorArmed = 0;
      refHeight = 0;
      LandingPhase = 0;
      initDone=0;
      note: Description:
          | -This state will wait for the host command to take off
    state Initialize
      entry:
      reset_offset_calc = 0;
      MotorArmed = 0;
      refHeight = 0;
      LandingPhase = 0;
      initDone=0;
      note: Description:
          | -Upon entry, this block will set the motor to NOT ARMED (turn off integrators in controller, set safety clamp of motors to OFF)
          | -Upon entry, set the refHeight to ZERO
          | -Upon entry, reset the offset calculation such that we can re-start the averaging block
      state Attitude_Convergence_Wait
        entry,during:
        Converge_Flag = checkConvergence(GyroOffset_Parameters);
      state converge = checkConvergence(Euler_Angles) [function]
      state Calculate_Attitude_Offset
        during:
        Offset_Accel_Current =Accel_Offset_Calculation(Offset_Parameters,reset_offset_calc);
        Offset_Gyro_Current =Gyro_Offset_Calculation(GyroOffset_Parameters,reset_offset_calc);
      state Done_Initialization
        entry:
      (default) -> Attitude_Convergence_Wait
      Attitude_Convergence_Wait -> Calculate_Attitude_Offset : [Converge_Flag==1 && after(0.1,sec)]
      Calculate_Attitude_Offset -> Calculate_Attitude_Offset [order 2] : [after(4,sec)]
          | {reset_offset_calc=1;
          | Offset_Accel = Offset_Accel_Current;
          | Offset_Gyro = Offset_Gyro_Current;}
      Calculate_Attitude_Offset -> Done_Initialization [order 1] : [reset_offset_calc == 1]
          | {Accel_Offset_Calculation(Offset_Parameters,reset_offset_calc);
          | Gyro_Offset_Calculation(GyroOffset_Parameters,reset_offset_calc);}
    state Controlled_Flight
      entry:
      LandingPhase = 0; refHeight = 0; MotorArmed =1;
      note: Description:
          | -Upon entry, this block will set the motor to ARMED (enable controller integrator and motor safetey unclamped)
          | -This block will command the AR Drone to fly up to a certain height using the variable refHeight
          | -The output of refHeight should be a function of desired Altitude. The most primitive assignment is to make refHeight = DesiredAltitude, this is comparable to giving the drone a step response. Alternate methods could be giving it a smooth trajectory to follow from the ground to that particular height
          |
          | -Below is an example of what it might look like
      state Altitude_Climb_Step1
        entry: refHeight = Desired_Altitude;
      state Altitude_Climb_Step2
        entry: refHeight = Desired_Altitude;
      state Altitude_Climb_Step3
        entry: refHeight = Desired_Altitude;
      state Altitude_Climb_Step5
        entry: refHeight = Desired_Altitude;
      (default) -> Altitude_Climb_Step1
      Altitude_Climb_Step1 -> Altitude_Climb_Step2 : after(5,sec)
      Altitude_Climb_Step2 -> Altitude_Climb_Step3 : after(5,sec)
      Altitude_Climb_Step3 -> Altitude_Climb_Step5 : after(5,sec)
    state Landing_Sequence
      entry:
      note: Description:
          | -Entry into this state will occur if
          | a) Battery drops to around 10.5-10.2 Volts (needs to be experimentally validated)
          | b) Entry condition is met from the user input
          | c) Attitude is out of bounds, ie: the quad rotor has tilted it's pitch to some uncontrollable angle such as 80 degrees
          |
          | Substate goals:
          | -Descend at a controllable rate and land safely
      state Climb_down_1
        entry: refHeight =1.3;
      state Climb_down_2
        entry:
        refHeight =0.5;
      state Climb_down_3
        entry: LandingPhase=1;
      (default) -> Climb_down_1 : {N=0;}
      Climb_down_2 -> Climb_down_3 : [UltraSound_Feedback(1)<=0.5 && after(0.1,sec)]
      Climb_down_1 -> Climb_down_2 : [UltraSound_Feedback(1)<=1.3 && after(0.1,sec)]
    state Landing_Terminate
      entry:
      MotorArmed =0;
      LandingPhase = 0;
      %Catch any last state action we need to do here
      note: Description:
          | This state is optional and might not be needed. Up to you if you think having an extra state for the landing phase might be useful.. if not, delete it and consolidate it into previous state
    (default) -> WaitForHost
    Landing_Terminate -> WaitForHost : [sum(MotorCmd)==0]
    WaitForHost -> Initialize : [ (hostCmd == Drone_StateModeType.Controlled_Flight)...
        |  &&...
        |  in(Fault_Check.BatteryFault_Check.BatteryNominal.Nominal) ]
    Controlled_Flight -> Landing_Terminate [order 2] : [in(Fault_Check.SafeOrientation_Check.UnsafeOrientation)]
    Controlled_Flight -> Landing_Sequence [order 1] : [(hostCmd == ...
        | Drone_StateModeType.Landing_Sequence)...
        | ||...
        |  in(Fault_Check.BatteryFault_Check.BatteryLow) ]
    Landing_Sequence -> Landing_Terminate : [sum(MotorCmd)==0]
    Done_Initialization -> Controlled_Flight
  state Flight_Controls [parallel]
    settings: executionOrder=2
    state Attitude_Command [parallel]
      entry, during:
      Attitude_Thrust = Attitude_Control(Desired_Attitude_deg,Euler_Angles,Angular_Velocity,MotorArmed);
      settings: executionOrder=1
    state Altitude_Command [parallel]
      entry, during:
      Altitude_Thrust = Altitude_Control(UltraSound_Feedback,refHeight);
      settings: executionOrder=2
    state MotorMixing_Command [parallel]
      entry, during:
      throttle = NominalThrust+EnableAltitudeCtrl*Altitude_Thrust;
      MotorCmd = Motor_Mixing(throttle,Attitude_Thrust,LandingPhase,MotorArmed);
      settings: executionOrder=3
  state deltaThrottle = Altitude_Control(HeightFeedback,refHeight) [function]
  state controls = Attitude_Control(Desired_Attitude_Deg,EulerAngle_Feedback_Deg,RateGyro_Feedback_Deg,Motor_Armed) [function]
  state MotorCommands = Motor_Mixing(throttle,RPYCmd,LandingPhase,Motor_Armed) [function]
  data: Euler_Angles function_input double size=3; converge function_output; OffsetMeasure function_input; Reset function_input; Y function_output; OffsetMeasure function_input; Reset function_input; Y function_output; HeightFeedback function_input double size=2; refHeight function_input double size=1; deltaThrottle function_output int16; Desired_Attitude_Deg function_input double size=3; EulerAngle_Feedback_Deg function_input double size=3; RateGyro_Feedback_Deg function_input double size=3; Motor_Armed function_input double size=1; controls function_output int16 size=3; throttle function_input int16 size=1; RPYCmd function_input int16 size=3; LandingPhase function_input double size=1; MotorCommands function_output; Motor_Armed function_input double size=1; hostCmd input Enum: Drone_StateModeType; Desired_Attitude_deg input size=3; UltraSound_Feedback input size=2; initDone local; refHeight output; MotorCmd output size=4; throttle local int16; deltaThrottle local; height local; Euler_Angles input; Angular_Velocity input; AccelVector_Input input; hoverHeight local; NominalThrust input; EnableAltitudeCtrl input; Drone_StateMode output Enum: Drone_StateModeType; Desired_Altitude input; Measured_Battery_Voltage input; Attitude_Thrust local; Altitude_Thrust local; Converge_Flag local; reset_offset_calc local; MotorArmed local; Offset_Accel data_store_memory; LandingPhase local; N local; Offset_Parameters input size=2; GyroOffset_Parameters input size=3; Offset_Gyro data_store_memory; Offset_Gyro_Current local; Offset_Value_Current local; Offset_Accel_Current local double; BatteryFault local; OrientationFault local; BatteryFault_Mode output Enum: BatteryFault_ModeType; SafeOrientation_Mode output Enum: SafeOrientation_ModeType
  data hostCmd settings: description=|
      | The hostCmd can take the values 0,1 and 2.
      | 
      | 0 - default state when the drone is powered up.
      | 1 - Takeoff
      | 2 - Landing
  data UltraSound_Feedback settings: description=Ultrasound Feedback will contain data on current height (cm) and altitude rate (cm/s)
  data initDone settings: description=A flag to check whether the calibration is done.
  data refHeight settings: description=Desired height at which the drone needs to hover.
  data NominalThrust settings: description=Nominal thrust input (approximately 60% duty cycle)
  data EnableAltitudeCtrl settings: description=A flag to enable the altitude controller
  function Y = Accel_Offset_Calculation(OffsetMeasure,Reset):
    | function Y = Accel_Offset_Calculation(OffsetMeasure,Reset)
    |  
    | %Compute running average while in this state. Assumed inputs
    | %are accelerometer offset values. These values are accumulated over time
    | %and divided by the total time increment to return an average values
    | Y = [0 0]';
    | persistent A_x_sum
    | persistent A_y_sum
    | persistent Tick
    | 
    | if(isempty(A_x_sum) || Reset==1)
    |     A_x_sum = 0;
    |     A_y_sum = 0;
    |     Tick = 1;
    |         
    | else
    |     
    |     Measure_X = OffsetMeasure(1);
    |     Measure_Y = OffsetMeasure(2);
    | 
    |     A_x_sum = A_x_sum + Measure_X;
    |     A_y_sum = A_y_sum + Measure_Y;
    | 
    | 
    |     Y = [A_x_sum A_y_sum]'./Tick;
    | 
    | 
    |     Tick = Tick + 1;
    | 
    | end
    | 
    | 
    | 
    | 
    | end
  function Y = Gyro_Offset_Calculation(OffsetMeasure,Reset):
    | function Y = Gyro_Offset_Calculation(OffsetMeasure,Reset)
    |  
    | %Compute running average while in this state. Assumed inputs
    | %are gyro offset values when drone is perfectly stationary on the ground. These values are accumulated over time
    | %and divided by the total time increment to return an average values
    | Y = [0 0 0]';
    | persistent A_x_sum
    | persistent A_y_sum
    | persistent A_z_sum
    | persistent Tick
    | 
    | if(isempty(A_x_sum) || Reset==1)
    |     A_x_sum = 0;
    |     A_y_sum = 0;
    |     A_z_sum = 0;
    | 
    |     Tick = 1;
    |         
    | else
    |     
    |     Measure_X = OffsetMeasure(1);
    |     Measure_Y = OffsetMeasure(2);
    |     Measure_Z = OffsetMeasure(3);
    | 
    |     A_x_sum = A_x_sum + Measure_X;
    |     A_y_sum = A_y_sum + Measure_Y;
    |     A_z_sum = A_z_sum + Measure_Z;
    | 
    | 
    |     Y = [A_x_sum A_y_sum A_z_sum]'./Tick;
    | 
    | 
    |     Tick = Tick + 1;
    | 
    | end
    | 
    | 
    | 
    | 
    | end

== matlab function New_Control_Law/Flight Controller/Supervisory Flight Controller/Attitude_Control/MATLAB Function ==
  data: error input; err_normalized output
function err_normalized = normalize_angle(error)
%#codegen

err_normalized = error;

% limit the yaw component to +/- 180 degrees
% if (error(3) > 180)    % Normalize to -180,180
%     err_normalized(3) = error(3) - 360;
% elseif(error(3) < -180)
%     err_normalized(3) = error(3) + 360;
% end

end

== matlab function New_Control_Law/Flight Controller/Supervisory Flight Controller/Motor_Mixing/RampDownInSpeed1 ==
  data: Cmd input; motorCmd output; stopCmd input
function motorCmd = fcn(Cmd,stopCmd)
%#codegen
persistent tempCmd;
if(isempty(tempCmd))
    tempCmd = ([0;0;0;0]);
end
if(stopCmd)
    tempCmd = tempCmd + ([1;1;1;1]*15/400);
    motorCmd = Cmd - tempCmd;
    
else
    tempCmd = ([0;0;0;0]);
    motorCmd = Cmd;
end

% if (motorCmd(1) <=0)
%         motorCmd = ([0;0;0;0]);
% end

%apply lower bounding
for i=1:4
    
if motorCmd(i)<0
    motorCmd(i) = 0;
end

end
